simulink model "Exp4A"  (R2015b)
settings: Solver=VariableStepAuto  StartTime=0.0  StopTime=0.7  RelTol=1e-5
libraries: dsparch4 x2, simulink x1
settings Model: Creator=mihai.ciobanu  LastModifiedBy=mihai.ciobanu
settings SolverCC: MaxConsecutiveMinStep=100

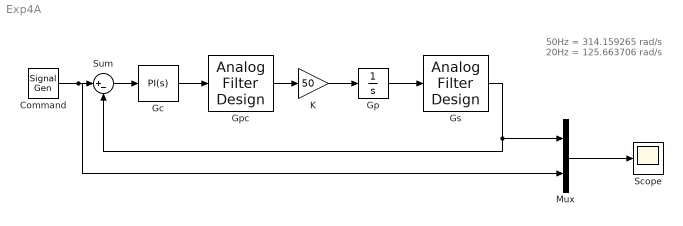
== system Exp4A ==
  note: 50Hz = 314.159265 rad/s
      | 20Hz = 125.663706 rad/s
  Command : SignalGenerator  WaveForm=square  Frequency=2
  Gc : simulink/Continuous/PID Controller  Controller=PI  TimeDomain=Continuous-time  SampleTime=-1  IntegratorMethod=Forward Euler  FilterMethod=Forward Euler  Form=Parallel  UseFilter=on  ControllerParametersSource=internal  P=1.5  I=30  D=0  N=100  InitialConditionSource=internal  InitialConditionForIntegrator=0  InitialConditionForFilter=0  ExternalReset=none  LimitOutput=off  UpperSaturationLimit=inf  LowerSaturationLimit=-inf  LinearizeAsGain=on  AntiWindupMode=none  Kb=1  TrackingMode=off  Kt=1  PParamMin=[]  PParamMax=[]  IParamMin=[]  IParamMax=[]  DParamMin=[]  DParamMax=[]  NParamMin=[]  NParamMax=[]  KbParamMin=[]  KbParamMax=[]  KtParamMin=[]  KtParamMax=[]  POutMin=[]  POutMax=[]  IOutMin=[]  IOutMax=[]  DOutMin=[]  DOutMax=[]  NOutMin=[]  NOutMax=[]  KbOutMin=[]  KbOutMax=[]  KtOutMin=[]  KtOutMax=[]  IntegratorOutMin=[]  IntegratorOutMax=[]  FilterOutMin=[]  FilterOutMax=[]  SumOutMin=[]  SumOutMax=[]  SumI1OutMin=[]  SumI1OutMax=[]  SumI2OutMin=[]  SumI2OutMax=[]  SumI3OutMin=[]  SumI3OutMax=[]  SumDOutMin=[]  SumDOutMax=[]  SaturationOutMin=[]  SaturationOutMax=[]  IntegratorContinuousStateAttributes=''  IntegratorStateMustResolveToSignalObject=off  IntegratorRTWStateStorageClass=Auto  FilterContinuousStateAttributes=''  FilterStateMustResolveToSignalObject=off  FilterRTWStateStorageClass=Auto  DifferentiatorICPrevScaledInput=0  DifferentiatorOutMin=[]  DifferentiatorOutMax=[]
  Gp : Integrator
  Gpc : dsparch4/Analog Filter Design  method=Butterworth  filttype=Lowpass  N=2  Wlo=314.159265  Whi=80  Rp=2  Rs=40
  Gs : dsparch4/Analog Filter Design  method=Butterworth  filttype=Lowpass  N=1  Wlo=125.663706  Whi=80  Rp=2  Rs=40
  K : Gain  Gain=50
  Mux : Mux  Inputs=2
  Scope : Scope
  Sum : Sum  Inputs=|+-
  wires:
  Sum/1 -> Gc/1
  Gc/1 -> Gpc/1
  Mux/1 -> Scope/1
  Command/1 -> Mux/2, Sum/1
  Gpc/1 -> K/1
  K/1 -> Gp/1
  Gp/1 -> Gs/1
  Gs/1 -> Mux/1, Sum/2
